simulink model "SimLinkLab1"  (R2019b)
settings: Solver=ode4  StartTime=0.0  StopTime=SimulationTime  FixedStep=1e-2  RelTol=1e-3
values from neighbouring files (symbols this model uses):
  FinalVoltage = 0    [ProgramLab1.m]
  InitialVoltage = 3    [ProgramLab1.m]
  K = 1/RC(i)    [ProgramLab1.m]
  StepTime = 5    [ProgramLab1.m]
  WPC = 0    [ProgramLab1.m]
settings Model: Creator=Illia Bannitsyn  LastModifiedBy=Illia Bannitsyn
settings DataIOCC: LimitDataPoints=on

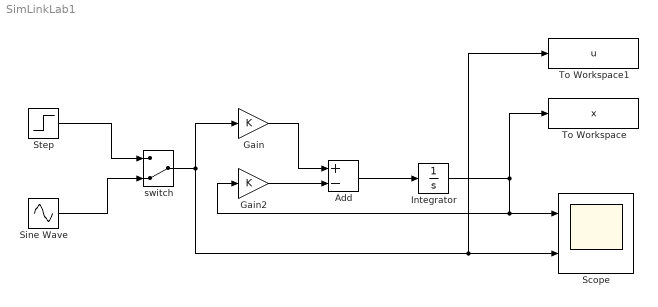
== system SimLinkLab1 ==
  Add : Sum  Inputs=+-
  Gain : Gain  Gain=K
  Gain2 : Gain  Gain=K
  Integrator : Integrator  InitialCondition=WPC
  Scope : Scope  NumInputPorts=2
  Sine Wave : Sin  Frequency=62  SampleTime=0
  Step : Step  Time=StepTime  Before=InitialVoltage  After=FinalVoltage  SampleTime=0  VectorParams1D=off
  To Workspace : ToWorkspace  VariableName=x  SampleTime=-1
      settings: MaxDataPoints=SimulationTime*100  Save2DSignal=2-D array (concatenate along first dimension)
  To Workspace1 : ToWorkspace  VariableName=u  SampleTime=-1
      settings: MaxDataPoints=SimulationTime*100  Save2DSignal=2-D array (concatenate along first dimension)
  switch : ManualSwitch  CurrentSetting=0
  wires:
  Sine Wave/1 -> switch/2
  Step/1 -> switch/1
  switch/1 -> Scope/2, To Workspace1/1, Gain/1
  Gain/1 -> Add/1
  Gain2/1 -> Add/2
  Add/1 -> Integrator/1
  Integrator/1 -> Scope/1, Gain2/1, To Workspace/1
